simulink library "PerformanceIndex"  (R2018a)
settings: Solver=VariableStepAuto  StartTime=0.0  StopTime=10.0  RelTol=1e-3
undefined symbols (not defined in the file or in its folder): ctrl, DiscIntNeverNeededParam
libraries: resettableTimer x2, meanEnergy x1, energyEstimate x1, powerEstimate x1
settings Model: Creator=mitch  LastModifiedBy=mitch

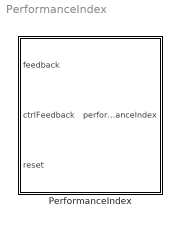
== system PerformanceIndex ==
  PerformanceIndex : Subsystem  Variant=on

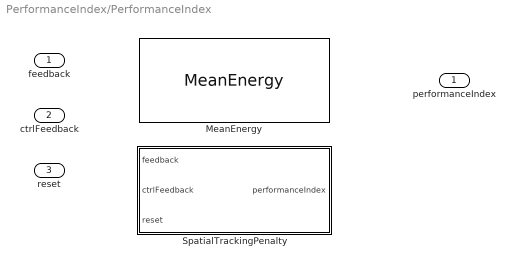
== system PerformanceIndex/PerformanceIndex ==
  feedback : Inport  OutDataTypeStr=Bus: busPlantFeedback
  ctrlFeedback : Inport  Port=2
  reset : Inport  Port=3  OutDataTypeStr=boolean
  MeanEnergy : meanEnergy/MeanEnergy  VariantControl=variantMeanEnergy
  SpatialTrackingPenalty : Subsystem  VariantControl=variantSpatialError
  performanceIndex : Outport

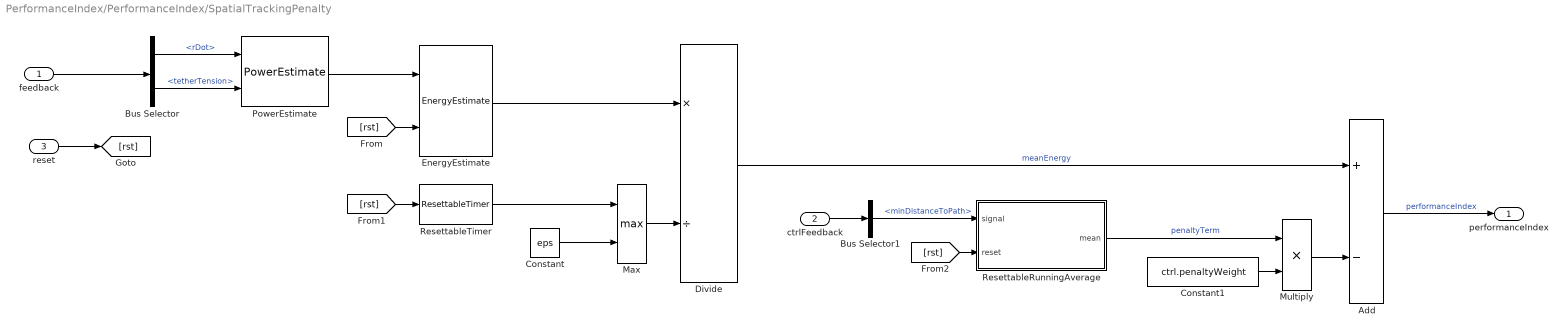
== system PerformanceIndex/PerformanceIndex/SpatialTrackingPenalty ==
  feedback : Inport
  ctrlFeedback : Inport  Port=2
  reset : Inport  Port=3
  Add : Sum  Inputs=+-
  Bus Selector : BusSelector  OutputSignals=rDot,tetherTension
  Bus Selector1 : BusSelector  OutputSignals=minDistanceToPath
  Constant : Constant  Value=eps
  Constant1 : Constant  Value=ctrl.penaltyWeight
  Divide : Product  Inputs=*/
  EnergyEstimate : energyEstimate/EnergyEstimate
  Max : MinMax  Function=max  Inputs=2
  Multiply : Product
  PowerEstimate : powerEstimate/PowerEstimate
  ResettableRunningAverage : Subsystem
  ResettableTimer : resettableTimer/ResettableTimer
  performanceIndex : Outport
  wires:
  Constant1/1 -> Multiply/2
  ResettableRunningAverage/1(mean) -> Multiply/1  "penaltyTerm"
  Multiply/1 -> Add/2
  Add/1 -> performanceIndex/1  "performanceIndex"
  [rst] -> ResettableRunningAverage/2(reset)
  [rst] -> ResettableTimer/1
  [rst] -> EnergyEstimate/2
  reset/1 -> [rst]
  Bus Selector1/1 -> ResettableRunningAverage/1(signal)  "<minDistanceToPath>"
  ctrlFeedback/1 -> Bus Selector1/1
  feedback/1 -> Bus Selector/1
  Constant/1 -> Max/2
  Bus Selector/2 -> PowerEstimate/2  "<tetherTension>"
  Max/1 -> Divide/2
  EnergyEstimate/1 -> Divide/1
  ResettableTimer/1 -> Max/1
  Divide/1 -> Add/1  "meanEnergy"
  Bus Selector/1 -> PowerEstimate/1  "<rDot>"
  PowerEstimate/1 -> EnergyEstimate/1

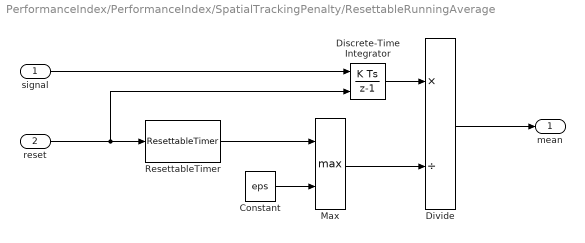
== system PerformanceIndex/PerformanceIndex/SpatialTrackingPenalty/ResettableRunningAverage ==
  signal : Inport
  reset : Inport  Port=2
  Constant : Constant  Value=eps
  Discrete-Time Integrator : DiscreteIntegrator  ExternalReset=rising  SampleTime=-1  ICPrevOutput=DiscIntNeverNeededParam  ICPrevScaledInput=DiscIntNeverNeededParam
  Divide : Product  Inputs=*/
  Max : MinMax  Function=max  Inputs=2
  ResettableTimer : resettableTimer/ResettableTimer
  mean : Outport
  wires:
  Divide/1 -> mean/1
  Discrete-Time Integrator/1 -> Divide/1
  Max/1 -> Divide/2
  Constant/1 -> Max/2
  ResettableTimer/1 -> Max/1
  signal/1 -> Discrete-Time Integrator/1
  reset/1 -> ResettableTimer/1, Discrete-Time Integrator/2
